simulink model "Furnace"  (R2020a)
settings: Solver=ode15s  StartTime=0  StopTime=27000  FixedStep=0.1  MaxStep=20  MinStep=1e-13  RelTol=1e-08  AbsTol=1e-09
undefined symbols (not defined in the file): agnostic_lqe_params, cont_reg, disturbance_type, F_aI_pid, F_aII_pid, input_type, k, lqe_params, LQR_params, LQRAgnostic_params, MPC_type, MPCDiscrete_function_parameters, MPCDiscreteAgnostic_function_parameters, MPCDiscreteDiffIntegralAgnostic_function_parameters, original_LQR_params, output_type, reg, single_butter_ss
libraries: simulink x35, cstblocks x10, mpclib x3
(part 6 of 8)

== system Furnace/Plant2/Boiler/Economizer ==
  T_fromHE : Inport
  T_fg : Inport  Port=2
  Fi_fg : Inport  Port=3
  F_w : Inport  Port=4
  Constant : Constant  Value=k.cp_fg
  Constant1 : Constant  Value=k.epsilon_ECO
  Constant2 : Constant  Value=k.eta_ECO
  Economizer : MATLAB Function  TreatAsAtomicUnit=on
  Transport Delay : TransportDelay  DelayTime=2  BufferSize=1024*2
  Transport Delay1 : TransportDelay  DelayTime=2  InitialOutput=k.T_amb  BufferSize=1024*2
  Transport Delay2 : TransportDelay  DelayTime=2  BufferSize=1024*2
  cp_water : Constant  Value=k.cp_water
  Q_ECO : Outport  VectorParamsAs1DForOutWhenUnconnected=off
  T_fg_out : Outport  Port=2  VectorParamsAs1DForOutWhenUnconnected=off
  Fi_fg_out : Outport  Port=3  VectorParamsAs1DForOutWhenUnconnected=off
  F_ECO : Outport  Port=4  VectorParamsAs1DForOutWhenUnconnected=off
  T_ECO2 : Outport  Port=5  VectorParamsAs1DForOutWhenUnconnected=off
  wires:
  Fi_fg/1 -> Fi_fg_out/1, Economizer/1(Fi_fg)
  T_fg/1 -> Economizer/4(T_fg2)
  T_fromHE/1 -> Economizer/3(T_ECO)
  Constant/1 -> Economizer/5(cp_fg)
  Constant1/1 -> Economizer/6(epsilon_ECO)
  Economizer/1(Q_ECO) -> Transport Delay/1
  Economizer/2(T_fg3) -> Transport Delay1/1
  F_w/1 -> Transport Delay2/1, Economizer/2(F_w)
  Transport Delay/1 -> Q_ECO/1
  Transport Delay1/1 -> T_fg_out/1
  Constant2/1 -> Economizer/7(eff_HE)
  cp_water/1 -> Economizer/8(cp_w)
  Economizer/3(T_ECO2) -> T_ECO2/1
  Transport Delay2/1 -> F_ECO/1

== system Furnace/Plant2/Boiler/Evaporator ==
  T_drum : Inport
  T_fg : Inport  Port=2
  Fi_fg : Inport  Port=3
  Constant : Constant  Value=k.cp_fg
  Constant1 : Constant  Value=k.epsilon_EVA
  Constant2 : Constant  Value=k.eff_HE
  Evaporator : MATLAB Function  TreatAsAtomicUnit=on
  Transport Delay : TransportDelay  DelayTime=5  InitialOutput=k.T_amb
  Q_EVA : Outport  VectorParamsAs1DForOutWhenUnconnected=off
  T_fg_out : Outport  Port=2  VectorParamsAs1DForOutWhenUnconnected=off
  Fi_fg_out : Outport  Port=3  VectorParamsAs1DForOutWhenUnconnected=off
  wires:
  T_drum/1 -> Evaporator/2(T_drum)
  Constant/1 -> Evaporator/4(cp_fg)
  Constant1/1 -> Evaporator/5(epsilon_EVA)
  Evaporator/1(Q_EVA) -> Q_EVA/1
  Evaporator/2(T_fg2) -> Transport Delay/1
  T_fg/1 -> Evaporator/3(T_fg1)
  Fi_fg/1 -> Fi_fg_out/1, Evaporator/1(Fi_fg)
  Transport Delay/1 -> T_fg_out/1
  Constant2/1 -> Evaporator/6(eff_HE)

== system Furnace/Plant2/Boiler/Super heater ==
  F_steam : Inport
  T_drum : Inport  Port=2
  T_fg : Inport  Port=3
  Fi_fg : Inport  Port=4
  Constant : Constant  Value=k.cp_fg
  Constant1 : Constant  Value=k.epsilon_SH
  Constant2 : Constant  Value=k.eff_HE
  Super heater : MATLAB Function  TreatAsAtomicUnit=on
  Transport Delay : TransportDelay  DelayTime=2  InitialOutput=k.T_amb
  Transport Delay1 : TransportDelay  DelayTime=2  InitialOutput=k.T_amb
  Transport Delay2 : TransportDelay  DelayTime=2
  Q_SH : Outport  VectorParamsAs1DForOutWhenUnconnected=off
  T_steam : Outport  Port=2  VectorParamsAs1DForOutWhenUnconnected=off
  T_fg_out : Outport  Port=3  VectorParamsAs1DForOutWhenUnconnected=off
  Fi_fg_out : Outport  Port=4  VectorParamsAs1DForOutWhenUnconnected=off
  F_SH : Outport  Port=5  VectorParamsAs1DForOutWhenUnconnected=off
  wires:
  F_steam/1 -> F_SH/1, Super heater/1(F_steam)
  T_drum/1 -> Super heater/3(T_drum)
  T_fg/1 -> Super heater/4(T_fg1)
  Constant/1 -> Super heater/5(cp_fg)
  Constant1/1 -> Super heater/6(epsilon_SH)
  Fi_fg/1 -> Fi_fg_out/1, Super heater/2(Fi_fg)
  Super heater/3(T_fg2) -> Transport Delay/1
  Super heater/2(T_steam) -> Transport Delay1/1
  Super heater/1(Q_SH) -> Transport Delay2/1
  Transport Delay/1 -> T_fg_out/1
  Transport Delay1/1 -> T_steam/1
  Transport Delay2/1 -> Q_SH/1
  Constant2/1 -> Super heater/7(eff_HE)

== system Furnace/Plant2/Grate/Q_rad ==
  T_rad : Inport
  T_w : Inport  Port=2
  A_rad : Inport  Port=3
  1/n_cell : Gain  Gain=1./k.n_cell
  "Power " : Constant  Value=4
  Product : Product
  T_rad^4 : Math  Operator=pow  SignedPower=on  OutputSignalType=real  SaturateOnIntegerOverflow=on
  T_w^4 : Math  Operator=pow  SignedPower=on  OutputSignalType=real  SaturateOnIntegerOverflow=on
  "alpha_gt " : Gain  Gain=k.alpha_gt
  epsilon : Gain  Gain=k.epsilon_gt
  sigma : Gain  Gain=k.sigma
  sum : Sum  Inputs=+-
  Q_rad : Outport  VectorParamsAs1DForOutWhenUnconnected=off
  wires:
  A_rad/1 -> 1/n_cell/1
  "Power "/1 -> T_w^4/2, T_rad^4/2
  sigma/1 -> Product/1
  epsilon/1 -> sum/1
  sum/1 -> sigma/1
  T_w^4/1 -> "alpha_gt "/1
  T_rad/1 -> T_rad^4/1
  T_w/1 -> T_w^4/1
  "alpha_gt "/1 -> sum/2
  Product/1 -> Q_rad/1
  T_rad^4/1 -> epsilon/1
  1/n_cell/1 -> Product/2

== system Furnace/Controller/MPC_subsystem/LQG_controller/Controller_battery ==
  x_lqe : Inport
  u_used : Inport  Port=2
  x_lqe_agnostic : Inport  Port=3
  ref : Inport  Port=4
  Block if not MPC : Gain  Gain=(reg.controller_type == ControllerType.MPC)|| (reg.controller_type == ControllerType.LQR)
  Constant : Constant  Value=MPC_type
  Controller selector 2 : MATLAB Function  TreatAsAtomicUnit=on
  Gain : Gain  Gain=(reg.controller_type == ControllerType.MPC)|| (reg.controller_type == ControllerType.LQR)
  Gain1 : Gain  Gain=(reg.controller_type == ControllerType.MPC)|| (reg.controller_type == ControllerType.LQR)
  LQR : Subsystem  Commented=on
  LQRAgnostic : Subsystem  Commented=on
  LQRDiffIntegral : Subsystem  Commented=on
  LQRDiffIntegralAgnostic : Subsystem  Commented=on
  MPCDiscrete : Subsystem  Commented=on
  MPCDiscreteAgnostic : Subsystem  Commented=on
  MPCDiscreteDiffIntegralAgnostic : Subsystem
  MPCPseudoDiscrete : Subsystem  Commented=on
  MPCPseudoDiscreteAgnostic : Subsystem  Commented=on
  Scope : Scope
  Scope1 : Scope
  Selector{,1..9} (10 alike) : Selector  InputPortWidth=4  IndexOptions=Index vector (dialog)  Indices=1:4  OutputSizes=1
  v_grate : Outport
  wires:
  MPCPseudoDiscrete/1(MPC_u) -> Selector1/1
  LQR/1(lqr_u) -> Selector2/1
  MPCDiscrete/1(u) -> Selector/1
  LQRDiffIntegral/1(lqr_u) -> Selector3/1
  Controller selector 2/1(signal) -> Selector5/1  "v_grate"
  u_used/1 -> Gain1/1
  ref/1 -> Gain/1
  x_lqe/1 -> Block if not MPC/1
  Selector/1 -> Controller selector 2/1(MPC_discrete)
  Selector1/1 -> Controller selector 2/2(MPC_pseudo_discrete)
  Selector2/1 -> Controller selector 2/3(LQR)
  Selector3/1 -> Controller selector 2/4(LQR_diff_integral)
  Constant/1 -> Controller selector 2/10(MPC_type)
  Selector5/1 -> Scope/1, v_grate/1
  MPCDiscreteAgnostic/1(u) -> Selector6/1
  LQRDiffIntegralAgnostic/1(lqr_u) -> Selector9/1
  LQRAgnostic/1(lqr_u) -> Selector8/1
  MPCPseudoDiscreteAgnostic/1(MPC_u) -> Selector7/1
  Selector6/1 -> Controller selector 2/5(Discrete_MPC_agnostic)
  Selector9/1 -> Controller selector 2/8(LQR_diff_integral_agnostic)
  Selector7/1 -> Controller selector 2/6(Pseudo_discrete_MPC_agnostic)
  Selector8/1 -> Controller selector 2/7(LQR_agnostic)
  Gain/1 -> MPCDiscreteDiffIntegralAgnostic/2(ref), MPCPseudoDiscreteAgnostic/2(ref), MPCDiscreteAgnostic/2(ref), MPCPseudoDiscrete/2(ref), MPCDiscrete/2(ref)
  Block if not MPC/1 -> Scope1/1, LQRDiffIntegral/1(x_hat), LQR/1(x_hat), MPCPseudoDiscrete/1(x), MPCDiscrete/1(x)
  x_lqe_agnostic/1 -> MPCPseudoDiscreteAgnostic/1(x), LQRAgnostic/1(x_hat), MPCDiscreteDiffIntegralAgnostic/1(x_hat_agnostic), LQRDiffIntegralAgnostic/1(x_hat_agnostic), MPCDiscreteAgnostic/1(x)
  MPCDiscreteDiffIntegralAgnostic/1(u) -> Selector4/1
  Selector4/1 -> Controller selector 2/9(MPCDiscreteDiffIntegralAgnostic)
  Gain1/1 -> MPCDiscreteDiffIntegralAgnostic/3(u_used), LQRDiffIntegralAgnostic/2(u_used), LQRDiffIntegral/2(u_used)

== system Furnace/Controller/MPC_subsystem/LQG_controller/Kalman filter battery ==
  note: Subsystem
  u_in : Inport
  v in : Inport  Port=2
  y : Inport  Port=3
  ref : Inport  Port=4
  Agnostic  lqr : Subsystem
  Assuming lqr : Subsystem
  Gain : Gain  Gain=(reg.controller_type == ControllerType.MPC)|| (reg.controller_type == ControllerType.LQR)
  Gain6 : Gain  Gain=lqe_params.integrator_direct_measurement_belief
  Gain7 : Gain  Gain=1-lqe_params.integrator_direct_measurement_belief
  Integrator : Integrator
  Manual Switch : ManualSwitch
  Scope : Scope
  Scope2 : Scope  NumInputPorts=2
  Scope4 : Scope
  Selector : Selector  InputPortWidth=3  IndexOptions=Index vector (dialog)  Indices=1:2  OutputSizes=1
  Selector1 : Selector  InputPortWidth=3  IndexOptions=Index vector (dialog)  Indices=1:3  OutputSizes=1
  Selector2 : Selector  InputPortWidth=3  IndexOptions=Index vector (dialog)  Indices=1:2  OutputSizes=1
  Selector3 : Selector  InputPortWidth=3  IndexOptions=Index vector (dialog)  Indices=1:2  OutputSizes=1
  Sum : Sum
  Sum1 : Sum  Inputs=-+|
  agnostic_anti_aliasing_filter : Subsystem
  anti_aliasing_filter : Subsystem
  y_MPC_hat : Outport
  Integrated_measurement_errors : Outport  Port=2
  x_hat_assuming : Outport  Port=3
  x_hat_agnostic : Outport  Port=4
  wires:
  y/1 -> Selector1/1  "Real measurement"
  Manual Switch/1 -> y_MPC_hat/1, Selector3/1, Gain7/1
  Integrator/1 -> Integrated_measurement_errors/1
  Assuming lqr/2(x_hat1) -> x_hat_assuming/1
  Agnostic  lqr/2(x_hat1) -> x_hat_agnostic/1
  Selector/1 -> Sum1/2
  Gain/1 -> Integrator/1
  Assuming lqr/1(y_hat) -> Manual Switch/1
  u_in/1 -> Agnostic  lqr/2(u), Assuming lqr/3(u)
  Gain7/1 -> Sum/1
  ref/1 -> Sum1/1
  Selector1/1 -> anti_aliasing_filter/1(In1), agnostic_anti_aliasing_filter/1(High_frequency_signal), Selector2/1, Gain6/1
  Sum1/1 -> Scope/1, Gain/1
  Selector2/1 -> Scope2/1
  v in/1 -> Assuming lqr/2(v in), Scope4/1
  Agnostic  lqr/1(y_hat) -> Manual Switch/2
  Sum/1 -> Selector/1
  Selector3/1 -> Scope2/2
  anti_aliasing_filter/1(Noisy y) -> Assuming lqr/1(Noisy y)
  Gain6/1 -> Sum/2
  agnostic_anti_aliasing_filter/1(filtered_signal) -> Agnostic  lqr/1(Noisy y)

== system Furnace/Deprecated, slow loop/Actuator dynamics/Secondary air/Flue gas fan ==
  note: rpm of impeller
  note: Shaft torque
  PID signal : Inport
  Alpha : Gain  Gain=k.alpha_est_aII.*100
  Constant : Constant  Value=k.omega_T_aII
  Divide : Product  Inputs=*/
  Efficiency : Gain  Gain=k.mu_eff
  Gain : Gain  Gain=1/(k.I_aII)
  Gain4 : Gain  Gain=60/(2*pi)
  Integrator : Integrator  InitialCondition=reg.F_aII_fan_model_int
  "Linear mapping from rpm to volume flow " : Gain  Gain=k.map_aII
  "Maksimum power " : Gain  Gain=k.Pmax_aII
  Plus2 : Sum  Inputs=+-
  Square : Math  Operator=square  SignedPower=on  SaturateOnIntegerOverflow=on
  Square1 : Math  Operator=square  SignedPower=on  SaturateOnIntegerOverflow=on
  Static pressure converter : Gain  Gain=k.alpha_est_aII*2*3.1415/k.map_aII
  Switch : Switch  Criteria=u2 > Threshold  Threshold=k.omega_T_aII
  Volume flow : Outport  VectorParamsAs1DForOutWhenUnconnected=off
  Pressure difference : Outport  Port=2  VectorParamsAs1DForOutWhenUnconnected=off
  Power consumption : Outport  Port=3  VectorParamsAs1DForOutWhenUnconnected=off
  wires:
  Integrator/1 -> Square/1, Gain4/1, Switch/2, Switch/1, Square1/1
  Divide/1 -> Plus2/1
  Gain4/1 -> "Linear mapping from rpm to volume flow "/1
  Square/1 -> Static pressure converter/1
  Efficiency/1 -> Pressure difference/1
  "Maksimum power "/1 -> Power consumption/1, Divide/1
  Static pressure converter/1 -> Efficiency/1
  Alpha/1 -> Plus2/2
  Square1/1 -> Alpha/1
  Gain/1 -> Integrator/1
  Plus2/1 -> Gain/1
  PID signal/1 -> "Maksimum power "/1
  "Linear mapping from rpm to volume flow "/1 -> Volume flow/1
  Switch/1 -> Divide/2
  Constant/1 -> Switch/3

== system Furnace/Deprecated, slow loop/Actuator dynamics/Waste and Primary air/Flue gas fan ==
  note: rpm of impeller
  note: Shaft torque
  PID signal : Inport
  Alpha : Gain  Gain=k.alpha_est_aII.*100
  Constant : Constant  Value=k.omega_T_aII
  Divide : Product  Inputs=*/
  Efficiency : Gain  Gain=k.mu_eff
  Gain : Gain  Gain=1/(k.I_aII)
  Gain4 : Gain  Gain=60/(2*pi)
  Integrator : Integrator  InitialCondition=reg.F_aI_fan_model_int
  "Linear mapping from rpm to volume flow " : Gain  Gain=k.map_aII
  "Maksimum power " : Gain  Gain=k.Pmax_aII
  Plus2 : Sum  Inputs=+-
  Square : Math  Operator=square  SignedPower=on  SaturateOnIntegerOverflow=on
  Square1 : Math  Operator=square  SignedPower=on  SaturateOnIntegerOverflow=on
  Static pressure converter : Gain  Gain=k.alpha_est_aII*2*3.1415/k.map_aII
  Switch : Switch  Criteria=u2 > Threshold  Threshold=k.omega_T_aII
  Volume flow : Outport  VectorParamsAs1DForOutWhenUnconnected=off
  Pressure difference : Outport  Port=2  VectorParamsAs1DForOutWhenUnconnected=off
  Power consumption : Outport  Port=3  VectorParamsAs1DForOutWhenUnconnected=off
  wires:
  Integrator/1 -> Square/1, Gain4/1, Switch/2, Switch/1, Square1/1
  Divide/1 -> Plus2/1
  Gain4/1 -> "Linear mapping from rpm to volume flow "/1
  Square/1 -> Static pressure converter/1
  Efficiency/1 -> Pressure difference/1
  "Maksimum power "/1 -> Power consumption/1, Divide/1
  Static pressure converter/1 -> Efficiency/1
  Alpha/1 -> Plus2/2
  Square1/1 -> Alpha/1
  Gain/1 -> Integrator/1
  Plus2/1 -> Gain/1
  PID signal/1 -> "Maksimum power "/1
  "Linear mapping from rpm to volume flow "/1 -> Volume flow/1
  Switch/1 -> Divide/2
  Constant/1 -> Switch/3

== system Furnace/Deprecated, slow loop/Contineous Summer student feedback (Not finished)/Secondary air/Flue gas fan ==
  note: Shaft torque
  note: rpm of impeller
  PID signal : Inport
  Alpha : Gain  Gain=k.alpha_est_aII.*100
  Constant : Constant  Value=k.omega_T_aII
  Divide : Product  Inputs=*/
  Efficiency : Gain  Gain=k.mu_eff
  Gain : Gain  Gain=1/(k.I_aII)
  Gain4 : Gain  Gain=60/(2*pi)
  Integrator : Integrator  InitialCondition=cont_reg.F_aII_fan_model_int
  "Linear mapping from rpm to volume flow " : Gain  Gain=k.map_aII
  "Maksimum power " : Gain  Gain=k.Pmax_aII
  Plus2 : Sum  Inputs=+-
  Square : Math  Operator=square  SignedPower=on  SaturateOnIntegerOverflow=on
  Square1 : Math  Operator=square  SignedPower=on  SaturateOnIntegerOverflow=on
  Static pressure converter : Gain  Gain=k.alpha_est_aII*2*3.1415/k.map_aII
  Switch : Switch  Criteria=u2 > Threshold  Threshold=k.omega_T_aII
  Volume flow : Outport  VectorParamsAs1DForOutWhenUnconnected=off
  Pressure difference : Outport  Port=2  VectorParamsAs1DForOutWhenUnconnected=off
  Power consumption : Outport  Port=3  VectorParamsAs1DForOutWhenUnconnected=off
  wires:
  Constant/1 -> Switch/3
  Switch/1 -> Divide/2
  "Linear mapping from rpm to volume flow "/1 -> Volume flow/1
  PID signal/1 -> "Maksimum power "/1
  Plus2/1 -> Gain/1
  Gain/1 -> Integrator/1
  Square1/1 -> Alpha/1
  Alpha/1 -> Plus2/2
  Static pressure converter/1 -> Efficiency/1
  "Maksimum power "/1 -> Divide/1, Power consumption/1
  Efficiency/1 -> Pressure difference/1
  Square/1 -> Static pressure converter/1
  Gain4/1 -> "Linear mapping from rpm to volume flow "/1
  Divide/1 -> Plus2/1
  Integrator/1 -> Square1/1, Switch/1, Switch/2, Gain4/1, Square/1

== system Furnace/Deprecated, slow loop/Contineous Summer student feedback (Not finished)/Waste and Primary air/Flue gas fan ==
  note: Shaft torque
  note: rpm of impeller
  PID signal : Inport
  Alpha : Gain  Gain=k.alpha_est_aII.*100
  Constant : Constant  Value=k.omega_T_aII
  Divide : Product  Inputs=*/
  Efficiency : Gain  Gain=k.mu_eff
  Gain : Gain  Gain=1/(k.I_aII)
  Gain4 : Gain  Gain=60/(2*pi)
  Integrator : Integrator  InitialCondition=cont_reg.F_aI_fan_model_int
  "Linear mapping from rpm to volume flow " : Gain  Gain=k.map_aII
  "Maksimum power " : Gain  Gain=k.Pmax_aII
  Plus2 : Sum  Inputs=+-
  Square : Math  Operator=square  SignedPower=on  SaturateOnIntegerOverflow=on
  Square1 : Math  Operator=square  SignedPower=on  SaturateOnIntegerOverflow=on
  Static pressure converter : Gain  Gain=k.alpha_est_aII*2*3.1415/k.map_aII
  Switch : Switch  Criteria=u2 > Threshold  Threshold=k.omega_T_aII
  Volume flow : Outport  VectorParamsAs1DForOutWhenUnconnected=off
  Pressure difference : Outport  Port=2  VectorParamsAs1DForOutWhenUnconnected=off
  Power consumption : Outport  Port=3  VectorParamsAs1DForOutWhenUnconnected=off
  wires:
  Constant/1 -> Switch/3
  Switch/1 -> Divide/2
  "Linear mapping from rpm to volume flow "/1 -> Volume flow/1
  PID signal/1 -> "Maksimum power "/1
  Plus2/1 -> Gain/1
  Gain/1 -> Integrator/1
  Square1/1 -> Alpha/1
  Alpha/1 -> Plus2/2
  Static pressure converter/1 -> Efficiency/1
  "Maksimum power "/1 -> Divide/1, Power consumption/1
  Efficiency/1 -> Pressure difference/1
  Square/1 -> Static pressure converter/1
  Gain4/1 -> "Linear mapping from rpm to volume flow "/1
  Divide/1 -> Plus2/1
  Integrator/1 -> Square1/1, Switch/1, Switch/2, Gain4/1, Square/1

== system Furnace/Deprecated, slow loop/Furnace/Boiler/Drum ==
  F_ECO : Inport
  Q_EVA : Inport  Port=2
  F_vap : Inport  Port=3
  T_ECO : Inport  Port=4
  Q_cleaning : Inport  Port=5
  Constant : Constant  Value=k.p_amb
  Constant1 : Constant  Value=k.T_amb
  Constant10 : Constant  Value=k.cp_fg
  Constant11 : Constant  Value=k.Mw_air
  Constant2 : Constant  Value=k.Mw_water
  Constant3 : Constant  Value=k.V_gas
  Constant5 : Constant  Value=k.cp_water
  Constant6 : Constant  Value=k.V_EVA
  Constant7 : Constant  Value=k.rho_water
  Constant8 : Constant  Value=k.M_steel
  Constant9 : Constant  Value=k.cp_steel
  "DIFF_Boiler " : MATLAB Function  TreatAsAtomicUnit=on
  DIFF_Boiler_2 : MATLAB Function  TreatAsAtomicUnit=on
  DIFF_Boiler_vap : MATLAB Function  TreatAsAtomicUnit=on
  Integrator : Integrator  InitialCondition=k.A_0
  Integrator1 : Integrator  InitialCondition=k.M_H2O
  Scope : Scope
  cp_w : Constant  Value=k.cp_water
  T_drum : Outport  VectorParamsAs1DForOutWhenUnconnected=off
  x_vap : Outport  Port=2  VectorParamsAs1DForOutWhenUnconnected=off
  p_drum : Outport  Port=3  PortDimensions=1  VectorParamsAs1DForOutWhenUnconnected=off
  wires:
  F_vap/1 -> "DIFF_Boiler "/3(F_SH)
  Q_EVA/1 -> "DIFF_Boiler "/1(Q_EVA)
  F_ECO/1 -> "DIFF_Boiler "/2(F_ECO)
  "DIFF_Boiler "/1(dA_dt) -> Integrator/1
  Integrator/1 -> DIFF_Boiler_2/1(A)
  DIFF_Boiler_vap/1(x_vap) -> x_vap/1
  DIFF_Boiler_2/2(p) -> DIFF_Boiler_vap/2(p), p_drum/1
  Constant/1 -> DIFF_Boiler_2/2(p_amb)
  Constant1/1 -> DIFF_Boiler_2/3(T_amb)
  Constant2/1 -> DIFF_Boiler_2/4(Mw_water), DIFF_Boiler_vap/3(Mw_water)
  Constant3/1 -> DIFF_Boiler_2/5(V_gas)
  Integrator1/1 -> DIFF_Boiler_vap/4(M_H2O), DIFF_Boiler_2/6(M_H2O)
  Constant5/1 -> DIFF_Boiler_2/7(cp_water)
  Constant6/1 -> DIFF_Boiler_2/8(V_EVA), DIFF_Boiler_vap/5(V_EVA)
  Constant7/1 -> DIFF_Boiler_2/9(rho_water), DIFF_Boiler_vap/6(rho_water)
  Constant8/1 -> DIFF_Boiler_2/10(M_steel)
  Constant9/1 -> DIFF_Boiler_2/11(cp_steel)
  Constant10/1 -> DIFF_Boiler_2/12(cp_fg)
  Constant11/1 -> DIFF_Boiler_2/13(Mw_air)
  T_ECO/1 -> "DIFF_Boiler "/4(T_ECO)
  DIFF_Boiler_2/1(T_drum) -> "DIFF_Boiler "/5(T_drum), DIFF_Boiler_vap/1(T_drum), T_drum/1
  Q_cleaning/1 -> "DIFF_Boiler "/6(Q_cleaning)
  cp_w/1 -> "DIFF_Boiler "/7(cp_water)
  "DIFF_Boiler "/2(dM_dt) -> Integrator1/1, Scope/1

== system Furnace/Deprecated, slow loop/Furnace/Boiler/Economizer ==
  T_fromHE : Inport
  T_fg : Inport  Port=2
  Fi_fg : Inport  Port=3
  F_w : Inport  Port=4
  Constant : Constant  Value=k.cp_fg
  Constant1 : Constant  Value=k.epsilon_ECO
  Constant2 : Constant  Value=k.eta_ECO
  Economizer : MATLAB Function  TreatAsAtomicUnit=on
  Transport Delay : TransportDelay  DelayTime=2
  Transport Delay1 : TransportDelay  DelayTime=2  InitialOutput=k.T_amb
  Transport Delay2 : TransportDelay  DelayTime=2
  cp_water : Constant  Value=k.cp_water
  Q_ECO : Outport  VectorParamsAs1DForOutWhenUnconnected=off
  T_fg_out : Outport  Port=2  VectorParamsAs1DForOutWhenUnconnected=off
  Fi_fg_out : Outport  Port=3  VectorParamsAs1DForOutWhenUnconnected=off
  F_ECO : Outport  Port=4  VectorParamsAs1DForOutWhenUnconnected=off
  T_ECO2 : Outport  Port=5  VectorParamsAs1DForOutWhenUnconnected=off
  wires:
  Fi_fg/1 -> Fi_fg_out/1, Economizer/1(Fi_fg)
  T_fg/1 -> Economizer/4(T_fg2)
  T_fromHE/1 -> Economizer/3(T_ECO)
  Constant/1 -> Economizer/5(cp_fg)
  Constant1/1 -> Economizer/6(epsilon_ECO)
  Economizer/1(Q_ECO) -> Transport Delay/1
  Economizer/2(T_fg3) -> Transport Delay1/1
  F_w/1 -> Transport Delay2/1, Economizer/2(F_w)
  Transport Delay/1 -> Q_ECO/1
  Transport Delay1/1 -> T_fg_out/1
  Constant2/1 -> Economizer/7(eff_HE)
  cp_water/1 -> Economizer/8(cp_w)
  Economizer/3(T_ECO2) -> T_ECO2/1
  Transport Delay2/1 -> F_ECO/1

== system Furnace/Deprecated, slow loop/Furnace/Boiler/Evaporator ==
  T_drum : Inport
  T_fg : Inport  Port=2
  Fi_fg : Inport  Port=3
  Constant : Constant  Value=k.cp_fg
  Constant1 : Constant  Value=k.epsilon_EVA
  Constant2 : Constant  Value=k.eff_HE
  Evaporator : MATLAB Function  TreatAsAtomicUnit=on
  Transport Delay : TransportDelay  DelayTime=5  InitialOutput=k.T_amb
  Q_EVA : Outport  VectorParamsAs1DForOutWhenUnconnected=off
  T_fg_out : Outport  Port=2  VectorParamsAs1DForOutWhenUnconnected=off
  Fi_fg_out : Outport  Port=3  VectorParamsAs1DForOutWhenUnconnected=off
  wires:
  T_drum/1 -> Evaporator/2(T_drum)
  Constant/1 -> Evaporator/4(cp_fg)
  Constant1/1 -> Evaporator/5(epsilon_EVA)
  Evaporator/1(Q_EVA) -> Q_EVA/1
  Evaporator/2(T_fg2) -> Transport Delay/1
  T_fg/1 -> Evaporator/3(T_fg1)
  Fi_fg/1 -> Fi_fg_out/1, Evaporator/1(Fi_fg)
  Transport Delay/1 -> T_fg_out/1
  Constant2/1 -> Evaporator/6(eff_HE)

== system Furnace/Deprecated, slow loop/Furnace/Boiler/Super heater ==
  F_steam : Inport
  T_drum : Inport  Port=2
  T_fg : Inport  Port=3
  Fi_fg : Inport  Port=4
  Constant : Constant  Value=k.cp_fg
  Constant1 : Constant  Value=k.epsilon_SH
  Constant2 : Constant  Value=k.eff_HE
  Super heater : MATLAB Function  TreatAsAtomicUnit=on
  Transport Delay : TransportDelay  DelayTime=2  InitialOutput=k.T_amb
  Transport Delay1 : TransportDelay  DelayTime=2  InitialOutput=k.T_amb
  Transport Delay2 : TransportDelay  DelayTime=2
  Q_SH : Outport  VectorParamsAs1DForOutWhenUnconnected=off
  T_steam : Outport  Port=2  VectorParamsAs1DForOutWhenUnconnected=off
  T_fg_out : Outport  Port=3  VectorParamsAs1DForOutWhenUnconnected=off
  Fi_fg_out : Outport  Port=4  VectorParamsAs1DForOutWhenUnconnected=off
  F_SH : Outport  Port=5  VectorParamsAs1DForOutWhenUnconnected=off
  wires:
  F_steam/1 -> F_SH/1, Super heater/1(F_steam)
  T_drum/1 -> Super heater/3(T_drum)
  T_fg/1 -> Super heater/4(T_fg1)
  Constant/1 -> Super heater/5(cp_fg)
  Constant1/1 -> Super heater/6(epsilon_SH)
  Fi_fg/1 -> Fi_fg_out/1, Super heater/2(Fi_fg)
  Super heater/3(T_fg2) -> Transport Delay/1
  Super heater/2(T_steam) -> Transport Delay1/1
  Super heater/1(Q_SH) -> Transport Delay2/1
  Transport Delay/1 -> T_fg_out/1
  Transport Delay1/1 -> T_steam/1
  Transport Delay2/1 -> Q_SH/1
  Constant2/1 -> Super heater/7(eff_HE)

== system Furnace/Deprecated, slow loop/Furnace/Grate/Q_rad ==
  T_rad : Inport
  T_w : Inport  Port=2
  A_rad : Inport  Port=3
  1/n_cell : Gain  Gain=1./k.n_cell
  "Power " : Constant  Value=4
  Product : Product
  T_rad^4 : Math  Operator=pow  SignedPower=on  OutputSignalType=real  SaturateOnIntegerOverflow=on
  T_w^4 : Math  Operator=pow  SignedPower=on  OutputSignalType=real  SaturateOnIntegerOverflow=on
  "alpha_gt " : Gain  Gain=k.alpha_gt
  epsilon : Gain  Gain=k.epsilon_gt
  sigma : Gain  Gain=k.sigma
  sum : Sum  Inputs=+-
  Q_rad : Outport  VectorParamsAs1DForOutWhenUnconnected=off
  wires:
  A_rad/1 -> 1/n_cell/1
  "Power "/1 -> T_w^4/2, T_rad^4/2
  sigma/1 -> Product/1
  epsilon/1 -> sum/1
  sum/1 -> sigma/1
  T_w^4/1 -> "alpha_gt "/1
  T_rad/1 -> T_rad^4/1
  T_w/1 -> T_w^4/1
  "alpha_gt "/1 -> sum/2
  Product/1 -> Q_rad/1
  T_rad^4/1 -> epsilon/1
  1/n_cell/1 -> Product/2

== system Furnace/Controller/MPC_subsystem/LQG_controller/Controller_battery/LQR ==
  x_hat : Inport
  LQR : Gain  Gain=-LQR_params.K_lqr  Multiplication=Matrix(K*u)
  LTI System1 : cstblocks/LTI System  sys=original_LQR_params.input_filter  IC=[]
  Scope1 : Scope
  Scope2 : Scope
  lqr_u : Outport
  wires:
  LQR/1 -> LTI System1/1  "lqr_u"
  x_hat/1 -> Scope1/1, LQR/1
  LTI System1/1 -> Scope2/1, lqr_u/1

== system Furnace/Controller/MPC_subsystem/LQG_controller/Controller_battery/LQRAgnostic ==
  x_hat : Inport
  LQR : Gain  Gain=-LQRAgnostic_params.K_lqr  Multiplication=Matrix(K*u)
  LTI System1 : cstblocks/LTI System  sys=original_LQRAgnostic_params.input_filter  IC=[]
  Scope1 : Scope
  Scope2 : Scope
  lqr_u : Outport
  wires:
  LTI System1/1 -> Scope2/1, lqr_u/1
  x_hat/1 -> LQR/1, Scope1/1
  LQR/1 -> LTI System1/1  "lqr_u"

== system Furnace/Controller/MPC_subsystem/LQG_controller/Controller_battery/LQRDiffIntegral ==
  x_hat : Inport
  u_used : Inport  Port=2
  Demux : Demux  Outputs=2
  Integrator : Integrator
  LQR1 : Gain  Gain=- LQRDiffIntegral_params.K_lqr(:,1:end-1)  Multiplication=Matrix(K*u)
  LQR2 : Gain  Gain=- LQRDiffIntegral_params.K_lqr(:,end:end)  Multiplication=Matrix(K*u)
  LTI System1 : cstblocks/LTI System  sys=original_LQRDiffIntegral_params.input_filter  IC=[]
  Scope{,1..3} (4 alike) : Scope
  Selector3 : Selector  InputPortWidth=4  IndexOptions=Index vector (dialog)  Indices=[1 3]  OutputSizes=1
  Sum2 : Sum  Inputs=-+
  Sum3 : Sum  Inputs=|++
  lqr_u : Outport
  wires:
  LQR1/1 -> Scope/1, Sum3/1  "lqr_u"
  u_used/1 -> Selector3/1
  Sum3/1 -> LTI System1/1  "lqr_u"
  Sum2/1 -> Integrator/1
  Demux/2 -> Sum2/2
  Integrator/1 -> Scope3/1, LQR2/1
  Selector3/1 -> Demux/1
  Demux/1 -> Sum2/1
  x_hat/1 -> Scope2/1, LQR1/1
  LQR2/1 -> Scope1/1, Sum3/2  "lqr_u"
  LTI System1/1 -> lqr_u/1

== system Furnace/Controller/MPC_subsystem/LQG_controller/Controller_battery/LQRDiffIntegralAgnostic ==
  x_hat_agnostic : Inport
  u_used : Inport  Port=2
  Demux : Demux  Outputs=2
  Integrator : Integrator
  LQR1 : Gain  Gain=- LQRDiffIntegralAgnostic_params.K_lqr(:,1:end-1)  Multiplication=Matrix(K*u)
  LQR2 : Gain  Gain=- LQRDiffIntegralAgnostic_params.K_lqr(:,end:end)  Multiplication=Matrix(K*u)
  LTI System1 : cstblocks/LTI System  sys=original_LQRDiffIntegralAgnostic_params.input_filter  IC=[]
  LTI System2 : cstblocks/LTI System  Commented=on  sys=original_diff_agnostic_mpc_params.input_filter  IC=[]
  Scope : Scope
  Scope1 : Scope
  Scope3 : Scope
  Selector3 : Selector  InputPortWidth=4  IndexOptions=Index vector (dialog)  Indices=[1 3]  OutputSizes=1
  Sum2 : Sum  Inputs=-+
  Sum3 : Sum  Inputs=|++
  lqr_u : Outport
  wires:
  LQR2/1 -> Sum3/2, Scope1/1  "lqr_u"
  Demux/1 -> Sum2/1
  Selector3/1 -> Demux/1
  Integrator/1 -> Scope3/1, LQR2/1
  Demux/2 -> Sum2/2
  Sum2/1 -> Integrator/1
  Sum3/1 -> LTI System1/1  "lqr_u"
  LQR1/1 -> Sum3/1, Scope/1  "lqr_u"
  LTI System1/1 -> lqr_u/1
  x_hat_agnostic/1 -> LQR1/1
  u_used/1 -> Selector3/1

== system Furnace/Controller/MPC_subsystem/LQG_controller/Controller_battery/MPCDiscrete ==
  x : Inport
  ref : Inport  Port=2
  LTI System1 : cstblocks/LTI System  sys=original_MPCDiscrete_params .input_filter  IC=[]
  MATLAB Function : MATLAB Function  TreatAsAtomicUnit=on
  Memory1 : Memory  InitialCondition=MPCDiscrete_function_parameters.iA  InheritSampleTime=on  LinearizeMemory=on  LinearizeAsDelay=on
  Memory4 : Memory  InheritSampleTime=on  LinearizeMemory=on  LinearizeAsDelay=on
  u : Outport
  wires:
  Memory4/1 -> MATLAB Function/3(u_prev)
  MATLAB Function/2(new_iA) -> Memory1/1
  MATLAB Function/1(u) -> LTI System1/1, Memory4/1
  Memory1/1 -> MATLAB Function/4(iA)
  ref/1 -> MATLAB Function/2(ref)
  x/1 -> MATLAB Function/1(x)
  LTI System1/1 -> u/1

== system Furnace/Controller/MPC_subsystem/LQG_controller/Controller_battery/MPCDiscreteAgnostic ==
  x : Inport
  ref : Inport  Port=2
  LTI System1 : cstblocks/LTI System  sys=original_MPCDiscreteAgnostic_params.input_filter  IC=[]
  MATLAB Function : MATLAB Function  TreatAsAtomicUnit=on
  Memory1 : Memory  InitialCondition=MPCDiscreteAgnostic_function_parameters.iA  InheritSampleTime=on  LinearizeMemory=on  LinearizeAsDelay=on
  Memory4 : Memory  InheritSampleTime=on  LinearizeMemory=on  LinearizeAsDelay=on
  u : Outport
  wires:
  LTI System1/1 -> u/1
  x/1 -> MATLAB Function/1(x)
  ref/1 -> MATLAB Function/2(ref)
  Memory1/1 -> MATLAB Function/4(iA)
  MATLAB Function/1(u) -> Memory4/1, LTI System1/1
  MATLAB Function/2(new_iA) -> Memory1/1
  Memory4/1 -> MATLAB Function/3(u_prev)

== system Furnace/Controller/MPC_subsystem/LQG_controller/Controller_battery/MPCDiscreteDiffIntegralAgnostic ==
  x_hat_agnostic : Inport
  ref : Inport  Port=2
  u_used : Inport  Port=3
  Demux : Demux  Outputs=2
  Ground : Ground
  Integrator : Integrator
  LTI System1 : cstblocks/LTI System  sys=original_MPCDiscreteAgnostic_params.input_filter  IC=[]
  MATLAB Function : MATLAB Function  TreatAsAtomicUnit=on
  Memory1 : Memory  InitialCondition=MPCDiscreteDiffIntegralAgnostic_function_parameters.iA  InheritSampleTime=on  LinearizeMemory=on  LinearizeAsDelay=on
  Memory4 : Memory  InheritSampleTime=on  LinearizeMemory=on  LinearizeAsDelay=on
  Selector10 : Selector  InputPortWidth=19  IndexOptions=Index vector (dialog)  Indices=1:19  OutputSizes=1
  Selector3 : Selector  InputPortWidth=4  IndexOptions=Index vector (dialog)  Indices=[1 3]  OutputSizes=1
  Sum2 : Sum  Inputs=-+
  Vector Concatenate : Concatenate
  Vector Concatenate1 : Concatenate
  u : Outport
  wires:
  LTI System1/1 -> u/1
  x_hat_agnostic/1 -> Vector Concatenate/1
  Vector Concatenate1/1 -> MATLAB Function/2(ref)
  Memory1/1 -> MATLAB Function/4(iA)
  MATLAB Function/1(u) -> Memory4/1, LTI System1/1
  MATLAB Function/2(new_iA) -> Memory1/1
  Memory4/1 -> MATLAB Function/3(u_prev)
  Selector3/1 -> Demux/1
  Demux/1 -> Sum2/1
  u_used/1 -> Selector3/1
  Demux/2 -> Sum2/2
  Sum2/1 -> Integrator/1
  Integrator/1 -> Vector Concatenate/2
  Vector Concatenate/1 -> Selector10/1
  Selector10/1 -> MATLAB Function/1(x)
  ref/1 -> Vector Concatenate1/1
  Ground/1 -> Vector Concatenate1/2

== system Furnace/Controller/MPC_subsystem/LQG_controller/Controller_battery/MPCPseudoDiscrete ==
  x : Inport
  ref : Inport  Port=2
  Cont mpc : MATLAB Function
  LTI System1 : cstblocks/LTI System  sys=original_MPCPseudoDiscrete_params.input_filter  IC=[]
  MPC_u : Outport
  wires:
  Cont mpc/1(u) -> LTI System1/1  "MPC_u"
  x/1 -> Cont mpc/1(x)
  ref/1 -> Cont mpc/2(ref)
  LTI System1/1 -> MPC_u/1

== system Furnace/Controller/MPC_subsystem/LQG_controller/Controller_battery/MPCPseudoDiscreteAgnostic ==
  x : Inport
  ref : Inport  Port=2
  Cont mpc : MATLAB Function
  LTI System1 : cstblocks/LTI System  sys=original_MPCPseudoDiscreteAgnostic_params.input_filter  IC=[]
  MPC_u : Outport
  wires:
  LTI System1/1 -> MPC_u/1
  ref/1 -> Cont mpc/2(ref)
  x/1 -> Cont mpc/1(x)
  Cont mpc/1(u) -> LTI System1/1  "MPC_u"

== system Furnace/Controller/MPC_subsystem/LQG_controller/Kalman filter battery/Agnostic  lqr ==
  Noisy y : Inport
  u : Inport  Port=2
  Gain2 : Gain  Gain=agnostic_lqe_params.K_lqe  Multiplication=Matrix(K*u)
  Gain4 : Gain  Gain=agnostic_lqe_params.observed_plant.C  Multiplication=Matrix(K*u)
  Gain5 : Gain  Gain=agnostic_lqe_params.observed_plant.D  Multiplication=Matrix(K*u)
  Scope : Scope
  Subsystem : Subsystem
  Sum2 : Sum  Inputs=+-
  Sum3 : Sum  Inputs=++|
  y_hat : Outport
  x_hat1 : Outport  Port=2
  wires:
  Noisy y/1 -> Sum2/1
  Gain5/1 -> Sum3/2
  Gain4/1 -> Sum3/1
  Sum2/1 -> Gain2/1, Scope/1
  u/1 -> Gain5/1, Subsystem/2(u)
  Sum3/1 -> y_hat/1, Sum2/2
  Subsystem/1(x_hat) -> Gain4/1, x_hat1/1
  Gain2/1 -> Subsystem/1(y_tilde)

== system Furnace/Controller/MPC_subsystem/LQG_controller/Kalman filter battery/Assuming lqr ==
  Noisy y : Inport
  v in : Inport  Port=2
  u : Inport  Port=3
  Gain2 : Gain  Gain=lqe_params.K_lqe  Multiplication=Matrix(K*u)
  Gain4 : Gain  Gain=lqe_params.observed_plant.C  Multiplication=Matrix(K*u)
  Gain5 : Gain  Gain=lqe_params.observed_plant.D  Multiplication=Matrix(K*u)
  Scope : Scope
  Subsystem : Subsystem
  Sum2 : Sum  Inputs=+-
  Sum3 : Sum  Inputs=++|
  y_hat : Outport
  x_hat1 : Outport  Port=2
  wires:
  Gain2/1 -> Subsystem/1(y_tilde)
  Subsystem/1(x_hat) -> x_hat1/1, Gain4/1
  Sum3/1 -> Sum2/2, y_hat/1
  u/1 -> Subsystem/3(u), Gain5/1
  Sum2/1 -> Scope/1, Gain2/1
  Gain4/1 -> Sum3/1
  Gain5/1 -> Sum3/2
  Noisy y/1 -> Sum2/1
  v in/1 -> Subsystem/2(v in)

== system Furnace/Controller/MPC_subsystem/LQG_controller/Kalman filter battery/agnostic_anti_aliasing_filter ==
  High_frequency_signal : Inport
  Gain1 : Gain  Gain=agnostic_lqe_params.anti_aliasing_filter.B  Multiplication=Matrix(K*u)
  Gain2 : Gain  Gain=agnostic_lqe_params.anti_aliasing_filter.A  Multiplication=Matrix(K*u)
  Gain3 : Gain  Gain=agnostic_lqe_params.anti_aliasing_filter.C  Multiplication=Matrix(K*u)
  Integrator1 : Integrator
  Sum2 : Sum  Inputs=|++
  filtered_signal : Outport
  wires:
  Integrator1/1 -> Gain2/1, Gain3/1
  Sum2/1 -> Integrator1/1
  High_frequency_signal/1 -> Gain1/1
  Gain3/1 -> filtered_signal/1
  Gain1/1 -> Sum2/1
  Gain2/1 -> Sum2/2

== system Furnace/Controller/MPC_subsystem/LQG_controller/Kalman filter battery/anti_aliasing_filter ==
  In1 : Inport
  Gain1 : Gain  Gain=lqe_params.anti_aliasing_filter.B  Multiplication=Matrix(K*u)
  Gain2 : Gain  Gain=lqe_params.anti_aliasing_filter.A  Multiplication=Matrix(K*u)
  Gain3 : Gain  Gain=lqe_params.anti_aliasing_filter.B  Multiplication=Matrix(K*u)
  Integrator1 : Integrator
  Sum2 : Sum  Inputs=|++
  Noisy y : Outport
  wires:
  Gain1/1 -> Sum2/1
  Gain2/1 -> Sum2/2
  Sum2/1 -> Integrator1/1
  Integrator1/1 -> Gain2/1, Gain3/1
  In1/1 -> Gain1/1
  Gain3/1 -> Noisy y/1

== system Furnace/Controller/MPC_subsystem/LQG_controller/Kalman filter battery/Agnostic  lqr/Subsystem ==
  y_tilde : Inport
  u : Inport  Port=2
  Gain7 : Gain  Gain=agnostic_lqe_params.observed_plant.A  Multiplication=Matrix(K*u)
  Gain9 : Gain  Gain=agnostic_lqe_params.observed_plant.B  Multiplication=Matrix(K*u)
  Integrator : Integrator
  Scope{,1..3} (4 alike) : Scope
  Sum : Sum  Inputs=|++
  Sum6 : Sum  Inputs=++|
  x_hat : Outport
  wires:
  u/1 -> Gain9/1
  y_tilde/1 -> Sum6/1, Scope/1
  Integrator/1 -> Scope3/1, Gain7/1, x_hat/1
  Sum6/1 -> Sum/1
  Sum/1 -> Integrator/1
  Gain7/1 -> Sum/2, Scope1/1
  Gain9/1 -> Scope2/1, Sum6/2

== system Furnace/Controller/MPC_subsystem/LQG_controller/Kalman filter battery/Assuming lqr/Subsystem ==
  y_tilde : Inport
  v in : Inport  Port=2
  u : Inport  Port=3
  Gain1 : Gain  Gain=lqe_params.G_lqe_measurements  Multiplication=Matrix(K*u)
  Gain7 : Gain  Gain=lqe_params.observed_plant.A  Multiplication=Matrix(K*u)
  Gain9 : Gain  Gain=lqe_params.observed_plant.B  Multiplication=Matrix(K*u)
  Integrator : Integrator
  Scope{,1..4} (5 alike) : Scope
  Sum : Sum  Inputs=|++
  Sum6 : Sum  Inputs=+++
  x_hat : Outport
  wires:
  Gain7/1 -> Scope1/1, Sum/2
  Sum/1 -> Integrator/1
  Gain9/1 -> Scope2/1, Sum6/2
  Sum6/1 -> Sum/1
  Integrator/1 -> x_hat/1, Gain7/1
  y_tilde/1 -> Sum6/1, Scope/1
  u/1 -> Gain9/1
  v in/1 -> Scope4/1, Gain1/1
  Gain1/1 -> Scope3/1, Sum6/3

== matlab function Furnace/Plant2/Gas cleaning systems/HeatEx 1 ==
  data: T_in input; T_out output; Fi_in input; T_damp input; epsilon input; Fi_out output; cp_fg input; Q output
function [T_out, Fi_out, Q] = fcn(T_in,Fi_in,  T_damp, epsilon,cp_fg)

% This block is already ready 

F_fg    = sum(Fi_in);
C_min   = cp_fg.*F_fg;
Q       = epsilon.*C_min.*(T_damp-T_in);
T_out   = T_in + Q./(cp_fg.*F_fg);
Fi_out  = Fi_in;

== matlab function Furnace/Plant2/Gas cleaning systems/HeatEx 2 ==
  data: T_in input; T_out output; Fi_fg input; Fi_fg output; T2_in input; Fi_fg2 input; epsilon input; eff input; T2_out output; Fi_fg2 output; cp_fg input; Q_loss output
function [T_out, Fi_fg,T2_out, Fi_fg2,Q_loss] = fcn(T_in,Fi_fg, T2_in,Fi_fg2, epsilon,eff,cp_fg)

% This block is already ready 

F_fg1   = sum(Fi_fg);
F_fg2   = sum(Fi_fg2);
C_min   = cp_fg.*min(F_fg1,F_fg2);
Q       = epsilon.*C_min.*(T2_in-T_in);
T_out   = T_in + Q./(cp_fg.*F_fg1);
T2_out  = T2_in- Q./eff./(cp_fg.*F_fg2);
Q_loss  = (1-eff).*Q./eff;

== matlab function Furnace/Plant2/Gas cleaning systems/HeatEx 3 ==
  data: T_in input; T_out output; Fi_fg input; T_damp input; Fi_fg output; Q output; epsilon input; cp_fg input
function [T_out, Fi_fg, Q] = fcn(T_in,Fi_fg,  T_damp,epsilon,cp_fg)

% This block is already ready 

F_fg    = sum(Fi_fg);
C_min   = cp_fg.*F_fg;
Q       = epsilon.*C_min.*(T_damp-T_in);
T_out   = T_in + Q./(cp_fg.*F_fg);

== matlab function Furnace/Plant2/Gas cleaning systems/HeatEx 4 ==
  data: T_in input; T_out output; Fi_fg input; Fi_fg output; T2_in input; Fi_fg2 input; epsilon input; T2_out output; Fi_fg2 output; cp_fg input
function [T_out, Fi_fg,T2_out, Fi_fg2] = fcn(T_in,Fi_fg, T2_in,Fi_fg2, epsilon,cp_fg)


F_fg1   = sum(Fi_fg);
F_fg2   = sum(Fi_fg2);
C_min   = cp_fg.*min(F_fg1,F_fg2);
Q       = epsilon.*C_min.*(T_in-T2_in);
T_out   = T_in - Q./(cp_fg.*F_fg1);
T2_out  = T2_in+ Q./(cp_fg.*F_fg2);

== matlab function Furnace/Plant2/Gas cleaning systems/SIGURD - Reaktor ==
  data: T_in input; T_out output; Fi_in input; F_flyash input; Fi_out output; F_kalk input; Mw_gas input; cp_fg input; F_solid output; F_H2O input
function [T_out, Fi_out, F_solid] = fcn(T_in,Fi_in, F_flyash,F_kalk,Mw_gas,cp_fg, F_H2O)

%%%%%%%%%%%%%%%%%%%%%%%%%%%%%%%%%%%%%%%%%%%%%%%%%%%%%%%%%%%%%%%%%%%%%%%%%%
% INPUTS:
% T_in      [K]         Temperature of the inlet flue gas
% Fi_in     [kg/s]      Vector of mass flow of the gas components
% F_kalk    [kg/s]      Mass flow of kalk
% Mw_gas    [kg/kmol]   Vector of molar masses of the gas components


T_out   = T_in;
Fi_out  = Fi_in;
% The total amount of solid particles equals the flow of flyashes that 
% follow the gas from the combustion chamber + the solid phase particles 
% that form in the reactor
F_solid = F_flyash + 0;

== matlab function Furnace/Plant2/Gas cleaning systems/SIGURD - SCR (Katalisator) ==
  data: T_in input; T_out output; Fi_fg input; Fi_fg output; F_NH3 input; Mw_gas input
function [T_out, Fi_fg] = fcn(T_in,Fi_fg, F_NH3,Mw_gas)

%%%%%%%%%%%%%%%%%%%%%%%%%%%%%%%%%%%%%%%%%%%%%%%%%%%%%%%%%%%%%%%%%%%%%%%%%%
% INPUTS:
% T_in      [K]         Temperature of the inlet flue gas
% Fi_in     [kg/s]      Vector of mass flow of the gas components
% F_kalk    [kg/s]      Mass flow of kalk
% Mw_gas    [kg/kmol]   Vector of molar masses of the gas components

T_out   = T_in;

== matlab function Furnace/Deprecated, slow loop/Furnace/Boiler/Super heater/Super heater ==
  data: Q_SH output; F_steam input; T_steam output size=1; Fi_fg input; T_drum input; T_fg1 input; cp_fg input; epsilon_SH input; T_fg2 output size=1; eff_HE input
function [Q_SH,T_steam,T_fg2] = CALC_Q_SH(F_steam,Fi_fg,T_drum,T_fg1,cp_fg,epsilon_SH,eff_HE)

% This function calculates the heat exchanged in the super heater

F_fg    = sum(Fi_fg); 

if F_steam == 0 
    T_steam = T_drum;
    T_fg2   = T_fg1;
    Q_SH    = 0;
else
    [~,T_sat,~,~,~,c_p]=SatWater;
    cp_steam= interp1(T_sat,c_p,T_drum,'linear','extrap');
    C_min   = min(cp_fg.*F_fg,cp_steam.*F_steam);
    Q_SH    = epsilon_SH.*C_min.*(T_fg1-T_drum);
    T_fg2   = T_fg1 - Q_SH./(cp_fg.*F_fg);
    T_steam =  T_drum + Q_SH./(cp_steam.*F_steam);
end
Q_SH        = Q_SH.*eff_HE;

== matlab function Furnace/Plant2/Gas cleaning systems/SIGURD - Scrubber ==
  data: T_in input; T_out output; Fi_in input; Fi_out output; F_NH3 input; Mw_gas input
function [T_out, Fi_out] = fcn(T_in,Fi_in, F_NH3,Mw_gas)

%%%%%%%%%%%%%%%%%%%%%%%%%%%%%%%%%%%%%%%%%%%%%%%%%%%%%%%%%%%%%%%%%%%%%%%%%%
% INPUTS:
% T_in      [K]         Temperature of the inlet flue gas
% Fi_in     [kg/s]      Vector of mass flow of the gas components
% F_kalk    [kg/s]      Mass flow of kalk
% Mw_gas    [kg/kmol]   Vector of molar masses of the gas components


T_out   = T_in;
Fi_out  = Fi_in;

== matlab function Furnace/Plant2/Gas cleaning systems/SIGURD - Slangefilter ==
  data: T_in input; T_out output; Fi_in input; Fi_solid input; F_kull input; Mw_gas input; Fi_out output; F_ashes output
function [T_out, Fi_out, F_ashes] = fcn(T_in,Fi_in,Fi_solid, F_kull,Mw_gas)


T_out   = T_in;
Fi_out  = Fi_in;
F_ashes = 0;

== matlab function Furnace/Plant2/Grate/Diff_Grate ==
  data: M_w input; dMw_dt_col output; T_w input; M_char input; Fi_w_in input; T_w_in input; F_aI input; T_aI input; Q_rad input; Q_burners input; Q_grate input; v_grate input; L input; Delta_H input; cp_w input; cp_steel input; M_steel_grate input; cp_fg input; Mw_w input; Mw_gas input; p_amb input; T_amb input; k_w input; k_grate input; W input; rho_w input; A_grate input; dTw_dt_col output; dMchar_dt_col output; F_fg_out output; F_flyash output; F_char_ash output; t input
function [dMw_dt_col,dTw_dt_col,dMchar_dt_col,F_fg_out,F_flyash,F_char_ash]= DIFF_Grate(M_w,T_w,M_char,Fi_w_in,T_w_in,F_aI,T_aI,Q_rad,Q_burners,Q_grate,v_grate,L,Delta_H,cp_w,cp_steel,M_steel_grate,cp_fg,Mw_w,Mw_gas,p_amb,T_amb,k_w,k_grate,W,rho_w,A_grate,t)

% This function calculates the mass and energy balance of the furnace. The
% furnace is treated as a one dimensional system, which is discretized in
% 'n_cell'-control volumes, in the direction of movement of the waste on 
% the grate.

%%%%%%%%%%%%%%%%%%%%%%%%%%%%%%%%%%%%%%%%%%%%%%%%%%%%%%%%%%%%%%%%%%%%%%%%%%
% Symbol        Units       Explanation
% INPUTS:
% M_w           [kg]        Mass of waste components in each cell of the furnace
% T_w           [K]         Temperature of waste in each cell ot the furnace
% M_char        [kg]        Mass char in each cell of the furnace
% Fi_w_in       [kg/s]      Waste component mass flows into the furnace (it
%                           enters the first cell of the furnace.
% T_w_in        [K]         Temperature of the waste entering the furnace
% F_aI          [kg/s]      Primary air component mass flows in each zone
%                           (there are 'n_zone'-zones)
% T_aI          [K]         Temperature of primary air (same in every zone)
% Q_rad         [W]         Radiative heat to each cell
% Q_burners     [W]         Toatal heat delivered by auxiliary burners
% Q_grate       [W]         Heat removed by grate cooling (only zones 1-3)
% k              -          Vector of constant parameters
% t             [s]         Time 
%%%%%%%%%%%%%%%%%%%%%%%%%%%%%%%%%%%%%%%%%%%%%%%%%%%%%%%%%%%%%%%%%%%%%%%%%%

%% SOLID WASTE 
T_w         = T_w';
M_char      = M_char';
n_cell      = length(T_w);
nc_w        = length(M_w)./n_cell;
M_w         = reshape(M_w,[nc_w,n_cell]);   % Transform vector M_w into a matrix
Mw_tot      = sum(M_w,1) + M_char;          % Total mass in each zone [kg]

%% GEOMETRTICAL GRID
n_zone      = length(F_aI);
L_zone      = L./n_zone;                    % [m]
L_cell      = L./n_cell;                    % [m]
n           = 50;
x_zone      = linspace(0,L,n*n_zone);
x_cell      = linspace(0,L,n*n_cell);
F_aI_x      = zeros(size(x_zone));
T_aI_x      = zeros(size(x_zone));
Q_grate_x   = zeros(size(x_zone));
if Q_burners > 0
    Q_grate = zeros(5,1);                   % No grate cooling when the burners are on
else 
    Q_grate = [Q_grate; 0; 0];              % There is no grate cooling in zone 4 and 5
end
for i=1:n_zone
    F_aI_x((i-1)*n+1:i*n)   = F_aI(i).*ones(1,n)./L_zone;
    T_aI_x((i-1)*n+1:i*n)   = T_aI.*ones(1,n);
    Q_grate_x((i-1)*n+1:i*n)= Q_grate(i).*ones(1,n)./L_zone;
end
F_aI_dx     = interp1(x_zone,F_aI_x,x_cell);
T_aI_dx     = interp1(x_zone,T_aI_x,x_cell);
Q_grate_dx  = interp1(x_zone,Q_grate_x,x_cell);
F_aI        = zeros(size(T_w));
T_aI        = zeros(size(T_w));
Q_grate     = zeros(size(T_w));

for i = 1:n_cell
    F_aI(1,i)   = trapz(x_cell((i-1)*n+1:i*n),F_aI_dx((i-1)*n+1:i*n));
    T_aI(1,i)   = trapz(x_cell((i-1)*n+1:i*n),F_aI_dx((i-1)*n+1:i*n).*T_aI_dx((i-1)*n+1:i*n))./F_aI(1,i);
    Q_grate(1,i)= trapz(x_cell((i-1)*n+1:i*n),Q_grate_dx((i-1)*n+1:i*n));
end
%% INPUTS 
% Flows and temperature of the waste leaving each cell
Fi_w_out    = zeros(size(M_w));
for i = 1:n_cell
    if t>=(i*L_cell/v_grate)
        Fi_w_out(:,i) = v_grate.*M_w(:,i)./L_cell;
    end
end
T_w_out     = [T_w(:,2:end) T_w(end)];
% Flows and temperature of the waste entering each cell
Fi_w_in     = [Fi_w_in, Fi_w_out(:,1:end-1)];
F_w_in      = sum(Fi_w_in,1);
T_w_in      = [T_w_in, T_w(:,1:end-1)];
% Primary air  
w_aI        = CALC_w_ha(T_amb,90,Mw_gas);
Fi_aI       = zeros(length(w_aI),length(T_w));
for i = 1:n_cell
    Fi_aI(:,i)  = w_aI(:,1).*F_aI(i);
end

%% CONDUCTION TERMS
h_w         = sum(M_w,1)./(rho_w.*W);  % the height of the waste is a function of the mass on the grate
A_w         = W.*h_w;
% Conduction heat through the waste layer
Q_cond_w_in = -k_w.*A_w.*(T_w-T_w_in)./L_cell;
Q_cond_w_out= [Q_cond_w_in(2:end), 0];
Q_cond_w_l = [0 -k_w.*A_w(2:end).*(T_w(2:end)-T_w_in(2:end))./L_cell];
Q_cond_w_r= [Q_cond_w_l(2:end), 0];
% Conduction heat through the metal grate
Q_cond_g_in = -k_grate.*A_grate.*(T_w-T_w_in)./L_cell;
Q_cond_g_out= -k_grate.*A_grate.*(T_w_out-T_w)./L_cell;
Q_cond_g_l = [0 -k_grate.*A_grate.*(T_w(2:end)-T_w_in(2:end))./L_cell];
Q_cond_g_r= [Q_cond_g_l(2:end), 0];
% Total conduction term for each cell 
Q_cond      = Q_cond_w_l - Q_cond_w_r + Q_cond_g_l - Q_cond_g_r;

%% BURNERS
Q_burn      = Q_burners./n_cell.*ones(1,n_cell);

%% REACTION RATES
R_w         = CALC_Rw_Char(M_w,T_w,M_char,Fi_aI,Mw_w,Mw_gas,p_amb);  

%% STATIONARY TOTAL GAS BALANCE
F_fg_out    = Fi_aI + R_w.gas;
F_flyash    = -R_w.waste_cons(end,:);

%% DIFFERENTIAL EQUATIONS
% Solid waste mass balance
F_reac      = R_w.waste_cons;
dMw_dt      = Fi_w_in - Fi_w_out + F_reac;
         
% Char mass balance
F_char_out  = v_grate.*M_char./L_cell;          % [kg/s]
F_char_in   = [0, F_char_out(:,1:end-1)];
F_char_reac = R_w.char + R_w.char_cons;
dMchar_dt   = F_char_in - F_char_out + F_char_reac;       

% Enargy balance
Delta_H_tot = -(R_w.waste_cons(1,:).*Delta_H(1) + ...
                sum(R_w.waste_cons(2:end-1,:)).*Delta_H(2) + ...
                R_w.char_cons.*Delta_H(3) );
dTw_dt      = 1./(cp_w.*Mw_tot +cp_steel.*M_steel_grate./n_cell).*((F_w_in+F_char_in).*cp_w.*(T_w_in-T_w)+F_aI.*cp_fg.*(T_aI-T_w)+...  	% Convective terms
              Delta_H_tot+...                                                                                   % Reaction term
              Q_rad' +...                                                                                       % Radiation term
              Q_cond +...                                                                                       % Conduction term
              Q_burn -...                                                                                       % Burners
              Q_grate);                                                                                         % Grate cooling
% Make outputs into colums
dMw_dt_col   = reshape(dMw_dt,[n_cell*nc_w,1]);
dMchar_dt_col= dMchar_dt';
dTw_dt_col   = dTw_dt';
% F_w_ash      = Fi_w_out(end+1-nc_w:end);
F_char_ash   = F_char_out(end);

== matlab function Furnace/Plant2/Turbine/Turbine ==
  data: T_SH input; F_SH input; p_drum input; W_el output; p_HP input; p_LP input; Q_turb output; eta_TURB input
function [W_el, Q_turb ]  = CALC_Turbine(T_SH,F_SH,p_drum,p_HP,p_LP,eta_TURB)

% This function calculates the heat exchanged in the economizer
[p_sat,T_sat,~,~,h_vap,c_p] = SatWater;
cp_vap  = interp1(p_sat,c_p,p_drum,'linear','extrap');
h_sat   = interp1(p_sat,h_vap,p_drum,'linear','extrap');
T_drum  = interp1(p_sat,T_sat,p_drum,'linear','extrap');
h_in    = h_sat + cp_vap.*(T_SH - T_drum);
h_HP    = interp1(p_sat,h_vap,p_HP,'linear','extrap');
% h_LP    = interp1(p_sat,h_vap,p_LP,'linear','extrap');
Q_in    = F_SH.*(h_in - h_HP);
W_el    = eta_TURB.*Q_in;
Q_turb  = (1-eta_TURB).*Q_in;

% % This function calculates the heat exchanged in the economizer
% [p_sat,T_sat,~,~,h_vap,c_p] = SatWater;
% cp_vap  = interp1(p_sat,c_p,p_drum,'linear','extrap');
% h_sat   = interp1(p_sat,h_vap,p_drum,'linear','extrap');
% T_drum  = interp1(p_sat,T_sat,p_drum,'linear','extrap');
% h_in    = h_sat + cp_vap.*(T_SH - T_drum);
% Q_in    = F_SH.*(cp_vap.*(T_SH-T_cond) - H_eva);
% eta_TURB= 32.74 - 0.026.*(T_toDH - 273.15) - 0.089.*(T_fromDH - 273.15);
% W_el    = eta_TURB.*Q_in./100;
% T_turb  = T_cond;

== matlab function Furnace/Controller/Controller selector  ==
  data: ab input; cascade input; signal output; mpc input; lqr input; controller_type input
function signal = ChooseController(ab, cascade, mpc, lqr,controller_type)
   
switch(controller_type)
        case ControllerType.AB
            signal = ab;
        case ControllerType.Cascade
            signal = cascade;
        case ControllerType.MPC
            signal = mpc;
        otherwise
            signal = lqr;
    end
end

== matlab function Furnace/Controller/Input  selector ==
  data: constant input; signal output; experimental input; controlled input; input_type input
function signal = ChooseSignal(constant, experimental, controlled, input_type)
    switch(input_type)
        case InputType.Experimental
            signal = experimental;
        case InputType.Controlled
            signal = controlled;
        otherwise
            signal = constant;
    end
end
